simulink model "Oven_System"  (R2016a)
settings: Solver=ode4  SolverMode=SingleTasking  StartTime=0.0  StopTime=60*50  FixedStep=1.0  RelTol=1e-3
values from neighbouring files (symbols this model uses):
  Area = windowArea + wallArea    (= 5.25)    [Controller.m]
  h_inf = 5.0    (= 5)    [Controller.m]
  M_cp = (M_Air*c_Air+M_SS*c_SS)    (= 7231.615)    [Controller.m]
  R_Cond = RWall*RWindow/(RWall + RWindow)    (= 9.980537951e-05)    [Controller.m]
  R_Conv = 1/(h_inf*Area)    (= 0.0380952380952)    [Controller.m]
libraries: simulink x1
settings Model: Creator=levi.hubbard  LastModifiedBy=levi.hubbard
settings DataIOCC: LimitDataPoints=on  SaveFormat=Array
settings OptimizationCC: BlockReduction=off  BooleanDataType=off
settings DebuggingCC: SaveWithParameterizedLinksMsg=none  UnderspecifiedInitializationDetection=Classic  MergeDetectMultiDrivingBlocksExec=none  SignalResolutionControl=TryResolveAllWithWarning
settings HardwareCC: ProdBitPerPointer=32  ProdLargestAtomicFloat=None  ProdIntDivRoundTo=Undefined  ProdEndianess=Unspecified  ProdWordSize=32  ProdHWDeviceType=32-bit Generic  TargetUnknown=on
settings ModelReferenceCC: PropagateSignalLabelsOutOfModel=off
settings ConfigComp: CovModelRefEnable=Off  CovSFcnEnable=off

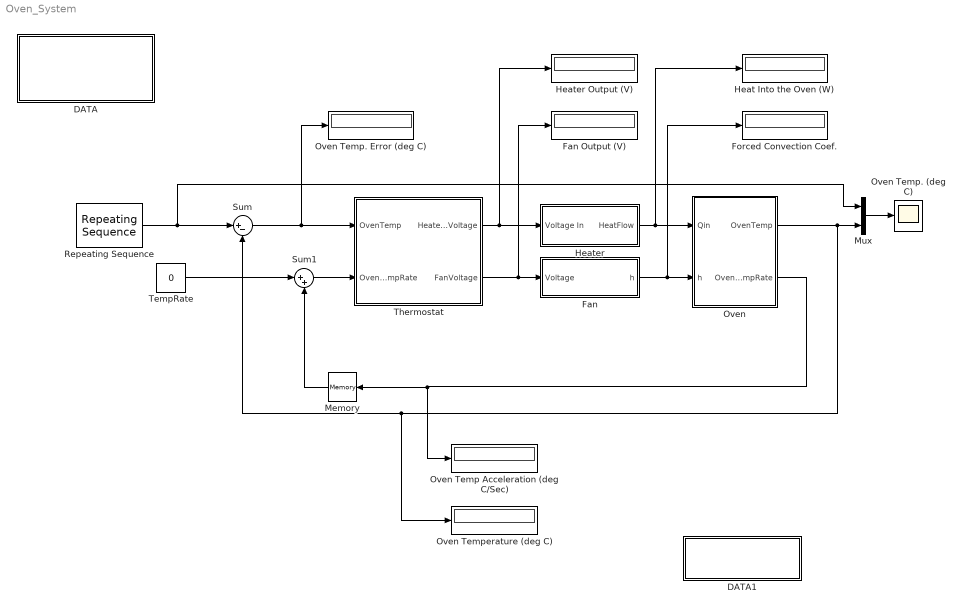
== system Oven_System ==
  DATA : Subsystem
      settings: OpenFcn=Controller
      mask Display: disp('Load System Params')
  DATA1 : Subsystem
      settings: OpenFcn=Graphs
      mask Display: disp('Display Graphs')
  Fan : Subsystem
  Fan Output (V) : Display
  Forced Convection Coef. : Display
  Heat Into the Oven (W) : Display
  "Heater " : Subsystem
  Heater Output (V) : Display
  Memory : Memory
  Mux : Mux  Inputs=2
  "Oven " : Subsystem
  Oven Temp Acceleration (deg C/Sec) : Display
  Oven Temp. (deg C) : Scope
  Oven Temp. Error (deg C) : Display
  Oven Temperature (deg C) : Display
  Repeating Sequence : simulink/Sources/Repeating Sequence  rep_seq_t=TimeForTemp  rep_seq_y=TempControl
  Sum : Sum  Inputs=|+-
  Sum1 : Sum  Inputs=|++
  TempRate : Constant  Value=0
  Thermostat : Subsystem
  wires:
  Repeating Sequence/1 -> Mux/1, Sum/1
  Sum/1 -> Oven Temp. Error (deg C)/1, Thermostat/1(OvenTemp)
  Fan/1(h) -> Forced Convection Coef./1, "Oven "/2(h)
  "Heater "/1(HeatFlow) -> Heat Into the Oven (W)/1, "Oven "/1(Qin)
  "Oven "/1(OvenTemp) -> Mux/2, Oven Temperature (deg C)/1, Sum/2
  Thermostat/1(HeaterVoltage) -> Heater Output (V)/1, "Heater "/1("Voltage In ")
  Thermostat/2(FanVoltage) -> Fan Output (V)/1, Fan/1(" Voltage ")
  TempRate/1 -> Sum1/1
  Sum1/1 -> Thermostat/2(OvenTampRate)
  "Oven "/2(OvenTempRate) -> Oven Temp Acceleration (deg C/Sec)/1, Memory/1
  Memory/1 -> Sum1/2
  Mux/1 -> Oven Temp. (deg C)/1

== system Oven_System/DATA ==

== system Oven_System/DATA1 ==

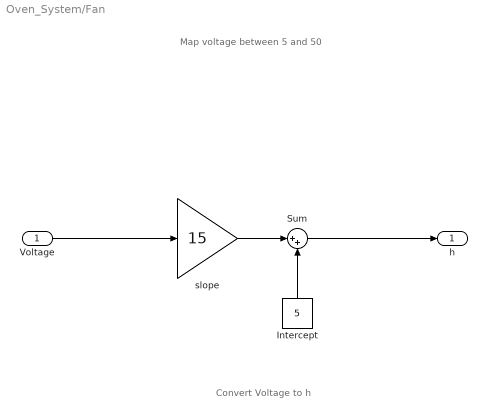
== system Oven_System/Fan ==
  note: Map voltage between 5 and 50
  note: Convert Voltage to h
  " Voltage " : Inport
  Intercept : Constant  Value=5
  Sum : Sum  Inputs=|++
  slope : Gain  Gain=15
  h : Outport
  wires:
  Sum/1 -> h/1
  " Voltage "/1 -> slope/1
  Intercept/1 -> Sum/2
  slope/1 -> Sum/1

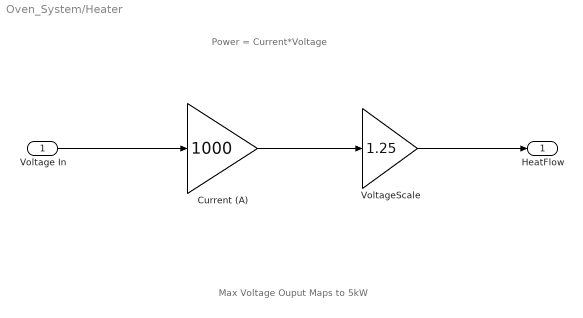
== system Oven_System/Heater  ==
  note: Max Voltage Ouput Maps to 5kW
  note: Power = Current*Voltage
  "Voltage In " : Inport
  Current (A) : Gain  Gain=1000
  VoltageScale : Gain  Gain=1.25
  HeatFlow : Outport
  wires:
  "Voltage In "/1 -> Current (A)/1
  Current (A)/1 -> VoltageScale/1
  VoltageScale/1 -> HeatFlow/1

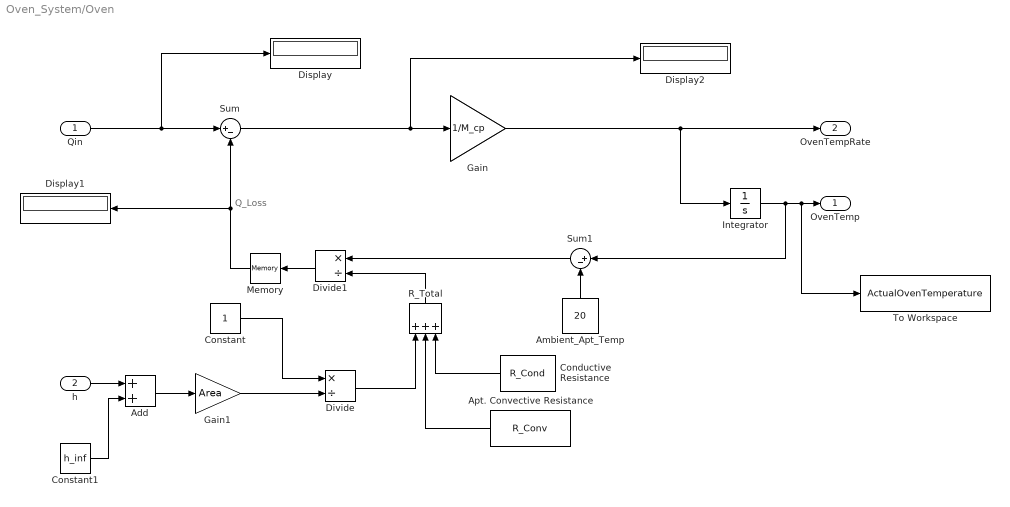
== system Oven_System/Oven  ==
  note: Q_Loss
  Qin : Inport
  h : Inport  Port=2
  " Apt. Convective Resistance" : Constant  Value=R_Conv
  Add : Sum
  Ambient_Apt_Temp : Constant  Value=20
  Conductive Resistance : Constant  Value=R_Cond
  Constant : Constant
  Constant1 : Constant  Value=h_inf
  Display : Display
  Display1 : Display
  Display2 : Display
  Divide : Product  Inputs=*/
  Divide1 : Product  Inputs=*/
  Gain : Gain  Gain=1/M_cp
  Gain1 : Gain  Gain=Area
  Integrator : Integrator
  Memory : Memory
  R_Total : Sum  Inputs=+++
  Sum : Sum  Inputs=|+-
  Sum1 : Sum  Inputs=|+-
  To Workspace : ToWorkspace  VariableName=ActualOvenTemperature  SampleTime=-1
  OvenTemp : Outport
  OvenTempRate : Outport  Port=2
  wires:
  Sum/1 -> Display2/1, Gain/1
  Gain/1 -> OvenTempRate/1, Integrator/1
  Ambient_Apt_Temp/1 -> Sum1/2
  Divide1/1 -> Memory/1
  Sum1/1 -> Divide1/1
  Integrator/1 -> To Workspace/1, OvenTemp/1, Sum1/1
  Conductive Resistance/1 -> R_Total/3
  " Apt. Convective Resistance"/1 -> R_Total/2
  Gain1/1 -> Divide/2
  Constant/1 -> Divide/1
  Divide/1 -> R_Total/1
  R_Total/1 -> Divide1/2
  h/1 -> Add/1
  Add/1 -> Gain1/1
  Constant1/1 -> Add/2
  Qin/1 -> Display/1, Sum/1
  Memory/1 -> Sum/2, Display1/1

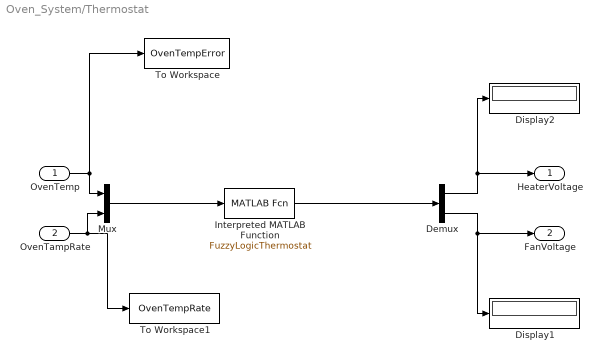
== system Oven_System/Thermostat ==
  OvenTemp : Inport
  OvenTampRate : Inport  Port=2
  Demux : Demux  Outputs=2
  Display1 : Display
  Display2 : Display
  Interpreted MATLAB Function : MATLABFcn  MATLABFcn=FuzzyLogicThermostat  OutputDimensions=2
  Mux : Mux  Inputs=2
  To Workspace : ToWorkspace  VariableName=OvenTempError  SampleTime=-1
  To Workspace1 : ToWorkspace  VariableName=OvenTempRate  SampleTime=-1
  HeaterVoltage : Outport
  FanVoltage : Outport  Port=2
  wires:
  OvenTampRate/1 -> To Workspace1/1, Mux/2
  OvenTemp/1 -> Mux/1, To Workspace/1
  Mux/1 -> Interpreted MATLAB Function/1
  Interpreted MATLAB Function/1 -> Demux/1
  Demux/1 -> HeaterVoltage/1, Display2/1
  Demux/2 -> Display1/1, FanVoltage/1
